simulink library "carnotUIBK"  (R2018b)
settings: Solver=VariableStepAuto  StartTime=0.0  StopTime=10.0  RelTol=1e-3  EnableMultiTasking=on
values from neighbouring files (symbols this model uses):
  A = 7*10*2    (= 140)    [theta_ground_v1.m]    (also in xlswrite1.m = num2cell(data))
  amb_factor = 1    [DOOR.m]    (also in WALL.m; WINDOW.m = 0)
  area = obj.width * obj.height    [DOOR.m]    (also in RES.m = []; ROOM.m = 0; THERMALZONE.m = area + room(kk).area; WALL.m = area - obj.doors(jj).calc_area())
  B = A/(0.5 * P)    (= 8.23529411765)    [theta_ground_v1.m]
  boundary = BOUNDARY()    [BUILDING.m]    (also in WALL.m = '')
  building = obj    [BUILDING.m]    (also in create_building_automatic.m = building.save(); ini_building_automatic.m = building.add_variant_hvac(building.variant_hvac, hvac); load_building_automatic.m = building.save())
  C = zeros(1,length(d)+1)    [CONSTRUCTION.m]    (also in DOOR.m = [0 0 0]; WALL.m = [0 0 0]; WINDOW.m = [0 0 0])
  control = 2    [GAIN.m]    (also in GAINS.m)
  cp = str2num(value)    [CONSTRUCTION.m]
  height = 0    [DOOR.m]    (also in ROOM.m; THERMALZONE.m; WALL.m; WINDOW.m)
  p = [timevec_weather weather(:,12)]    [BOUNDARY.m]    (also in WEATHER.m = 0; init_carnotUIBK.m = cell2mat(carnotUIBKpaths(i,2)))
  rho = str2num(value)    [CONSTRUCTION.m]    (also in theta_ground_v1.m = 2000)
  type = 1    [CONSTRUCTION.m]    (also in GAINS.m = raw_moisture{ii,3}; STRUCTURE.m = 0)
  view_factor = 1    [DOOR.m]    (also in WINDOW.m = 0)
  wall = []    [ROOM.m]
  z = obj.Z    [WALL.m]    (also in theta_ground_v1.m = 0)
  zone = obj.zone(ind)    [THERMALZONE.m]
undefined symbols (not defined in the file or in its folder): const, Dd, get_building, pos, Qdot_C, Qdot_H, Qdot_I_electricity, Qdot_I_light, Qdot_I_person, Qdot_S, Qdot_T_ground, Qdot_T_neighbour, Qdot_T_opaque, Qdot_T_window, Qdot_V_infiltration, Qdot_V_mech, Qdot_V_window, r_frame, solar_ratio, solar_ratio1, solar_ratio2, Tc, Tr, Ts, Uvalue, wallsurface, window, window_height, window_heigth, window_width, windowsurface, x_CO2, x_H2O, x_VOC
libraries: carnot x104, simulink x16, $bdroot x16, simulink_extras x14
(part 10 of 12)

== system carnotUIBK/wall_intersection/hygrothermal model/alpha_i2/alpha_i_horizontal ==
  note: (W/m^2)
  note: Convective and radiative heat transfer at the INDOOR SURFACE of a VERTICAL OUTER WALL
  note: CONVENTION:
      | Qdot > 0 and qdots < 0, if Ts > T (heat flows from wall surface to room node),
      | Qdot < 0 and qdots > 0, if Ts < T (heat flows from room node to wall surface).
  note: s: surface
      | c: convective
      | r: radiative
  note: dynamic, convective heat transfer coefficients according to: Glück B.: Wärmeübergangskoeffizienten an thermisch aktiven Bauteiloberflächen
      | und der Übergang zu Basiskennlinien für die Wärmestromdichte; gi Gesundheits-Ingenieur; 128. Jahrgang 2007, Heft 1, Seiten 1-10
  Ts : Inport
  AIB : Inport  Port=2
  Qdot sol : Inport  Port=3
  phis : Inport  Port=4
  1/wallsurface : Gain  Gain=1/wallsurface  SaturateOnIntegerOverflow=on  OutDataTypeStr=Inherit: Same as input  ParamDataTypeStr=Inherit: Same as input
  Add : Sum  Inputs=+-
  Bus Selector : BusSelector  OutputSignals=Tc,Tr,p,x_H2O
  Constant3 : Constant  Value=zeros(1,2)
  Constant4 : Constant  Value=zeros(1,4)
  Constant5 : Constant  Value=zeros(1,9)
  Fcn : Fcn  Expr=1.6*(abs(u(1)-u(2)))^0.3
  Fcn1 : Fcn  Expr=(273.15+u(1))^4-(273.15+u(2))^4
  Gain2 : Gain  Gain=0.01
  Mux : Mux  Inputs=2
  Mux2 : Mux  Inputs=2
  Mux3 : Mux  Inputs=2
  Mux4 : Mux  Inputs=[2 2 1 4 1 9]
  Product : Product  SaturateOnIntegerOverflow=on  RndMeth=Zero  InputSameDT=on  OutDataTypeStr=Inherit: Same as first input
  Product1 : Product  SaturateOnIntegerOverflow=on  RndMeth=Zero  InputSameDT=on  OutDataTypeStr=Inherit: Same as first input
  Product2 : Product  RndMeth=Zero
  Product3 : Product  RndMeth=Zero
  Product4 : Product  SaturateOnIntegerOverflow=on  RndMeth=Zero  InputSameDT=on  OutDataTypeStr=Inherit: Same as first input
  Sum : Sum  Inputs=+-  SaturateOnIntegerOverflow=on  InputSameDT=on  OutDataTypeStr=Inherit: Same as first input
  Sum of Elements : Sum  Inputs=+
  Sum2 : Sum  Inputs=+--  SaturateOnIntegerOverflow=on  InputSameDT=on  OutDataTypeStr=Inherit: Same as first input
  Switch : Switch  Criteria=u2 > Threshold
  emission_in : Gain  Gain=emission_in  SaturateOnIntegerOverflow=on  OutDataTypeStr=Inherit: Same as input  ParamDataTypeStr=Inherit: Same as input
  lewis : Gain  Gain=0.000000007  SaturateOnIntegerOverflow=on  OutDataTypeStr=Inherit: Same as input  ParamDataTypeStr=Inherit: Same as input
  nomassflow : Constant  Value=0
  ps_l : Fcn  Expr=610.0*exp(17.08*(u)/(234.2+(u)))
  ps_s_l : Fcn  Expr=610.0*exp(17.08*(u)/(234.2+(u)))
  sigma : Constant  Value=5.67e-8
  view_factor : Gain  Gain=view_factor  SaturateOnIntegerOverflow=on  OutDataTypeStr=Inherit: Same as input  ParamDataTypeStr=Inherit: Same as input
  wallsurface : Gain  Gain=wallsurface  SaturateOnIntegerOverflow=on  OutDataTypeStr=Inherit: Same as input  ParamDataTypeStr=Inherit: Same as input
  wallsurface1 : Gain  Gain=wallsurface  SaturateOnIntegerOverflow=on  OutDataTypeStr=Inherit: Same as input  ParamDataTypeStr=Inherit: Same as input
  x2RelHum_UIBK : carnot/Basic/Material_Properties/x2RelHum
  qdots : Outport  InitialOutput=0
  "[S]" : Outport  Port=2  InitialOutput=0
  alpha_c : Outport  Port=3  InitialOutput=0
  phi_i_1/100 : Outport  Port=4  InitialOutput=0
  wires:
  nomassflow/1 -> Switch/3
  Switch/1 -> Mux4/3
  wallsurface1/1 -> Switch/1
  view_factor/1 -> Product/1
  phis/1 -> Product3/1, Switch/2
  Product2/1 -> Add/2
  Product3/1 -> Add/1
  ps_s_l/1 -> Product3/2
  ps_l/1 -> Product2/2
  lewis/1 -> wallsurface1/1
  Gain2/1 -> Product2/1, phi_i_1/100/1
  Bus Selector/4 -> x2RelHum_UIBK/3  "<x_H2O>"
  Bus Selector/3 -> x2RelHum_UIBK/2  "<p>"
  x2RelHum_UIBK/1 -> Gain2/1
  Fcn1/1 -> Product/2
  Mux3/1 -> Fcn1/1
  sigma/1 -> emission_in/1
  Mux4/1 -> "[S]"/1
  Sum2/1 -> qdots/1
  AIB/1 -> Bus Selector/1
  Bus Selector/1 -> Sum/2, Mux2/2, x2RelHum_UIBK/1, ps_l/1  "<Tc>"
  emission_in/1 -> view_factor/1
  Product/1 -> Sum2/3, Mux/2  "qdotr"
  Mux/1 -> wallsurface/1
  Ts/1 -> Sum/1, ps_s_l/1, Mux3/1, Mux2/1  "Ts"
  Sum/1 -> Product1/1  "dTc"
  Bus Selector/2 -> Mux3/2  "<Tr>"
  Mux2/1 -> Fcn/1
  Product1/1 -> Mux/1, Sum2/2  "qdotc"
  Fcn/1 -> Product4/1, alpha_c/1, Product1/2  "hc"
  wallsurface/1 -> Sum of Elements/1, Mux4/1  "[Qdotc, Qdotr]"
  Qdot sol/1 -> 1/wallsurface/1
  1/wallsurface/1 -> Sum2/1
  Constant5/1 -> Mux4/6
  Constant4/1 -> Mux4/4
  Constant3/1 -> Mux4/2
  Sum of Elements/1 -> Mux4/5
  Add/1 -> Product4/2
  Product4/1 -> lewis/1

== system carnotUIBK/wall_intersection/hygrothermal model/alpha_i2/alpha_i_up ==
  note: (W/m^2)
  note: Convective and radiative heat transfer at the INDOOR SURFACE of a ceiling
  note: CONVENTION:
      | Qdot > 0 and qdots < 0, if Ts > T (heat flows from wall surface to room node),
      | Qdot < 0 and qdots > 0, if Ts < T (heat flows from room node to wall surface).
  note: s: surface
      | c: convective
      | r: radiative
  note: dynamic, convective heat transfer coefficients according to: Glück B.: Wärmeübergangskoeffizienten an thermisch aktiven Bauteiloberflächen
      | und der Übergang zu Basiskennlinien für die Wärmestromdichte; gi Gesundheits-Ingenieur; 128. Jahrgang 2007, Heft 1, Seiten 1-10
  Ts : Inport
  AIB : Inport  Port=2
  Qdot sol : Inport  Port=3
  phis : Inport  Port=4
  1/wallsurface : Gain  Gain=1/wallsurface  SaturateOnIntegerOverflow=on  OutDataTypeStr=Inherit: Same as input  ParamDataTypeStr=Inherit: Same as input
  Add : Sum  Inputs=+-
  Bus Selector : BusSelector  OutputSignals=Tc,Tr,p,x_H2O
  Constant3 : Constant  Value=zeros(1,2)
  Constant4 : Constant  Value=zeros(1,4)
  Constant5 : Constant  Value=zeros(1,9)
  Fcn1 : Fcn  Expr=(273.15+u(1))^4-(273.15+u(2))^4
  Gain2 : Gain  Gain=0.01
  Mux : Mux  Inputs=2
  Mux2 : Mux  Inputs=2
  Mux3 : Mux  Inputs=2
  Mux4 : Mux  Inputs=[2 2 1 4 1 9]
  Product : Product  SaturateOnIntegerOverflow=on  RndMeth=Zero  InputSameDT=on  OutDataTypeStr=Inherit: Same as first input
  Product1 : Product  SaturateOnIntegerOverflow=on  RndMeth=Zero  InputSameDT=on  OutDataTypeStr=Inherit: Same as first input
  Product2 : Product  RndMeth=Zero
  Product3 : Product  RndMeth=Zero
  Product4 : Product  SaturateOnIntegerOverflow=on  RndMeth=Zero  InputSameDT=on  OutDataTypeStr=Inherit: Same as first input
  Sum : Sum  Inputs=+-  SaturateOnIntegerOverflow=on  InputSameDT=on  OutDataTypeStr=Inherit: Same as first input
  Sum of Elements : Sum  Inputs=+
  Sum2 : Sum  Inputs=+--  SaturateOnIntegerOverflow=on  InputSameDT=on  OutDataTypeStr=Inherit: Same as first input
  Switch : Switch  Criteria=u2 > Threshold
  Switch1 : Switch
  emission_in : Gain  Gain=emission_in  SaturateOnIntegerOverflow=on  OutDataTypeStr=Inherit: Same as input  ParamDataTypeStr=Inherit: Same as input
  heat flux downwards : Fcn  Expr=0.54*(abs(u(1)-u(2))^0.31)
  heat flux upwards : Fcn  Expr=2*(abs(u(1)-u(2))^0.31)
  lewis : Gain  Gain=0.000000007  SaturateOnIntegerOverflow=on  OutDataTypeStr=Inherit: Same as input  ParamDataTypeStr=Inherit: Same as input
  nomassflow : Constant  Value=0
  ps_l : Fcn  Expr=610.0*exp(17.08*(u)/(234.2+(u)))
  ps_s_l : Fcn  Expr=610.0*exp(17.08*(u)/(234.2+(u)))
  sigma : Constant  Value=5.67e-8
  view_factor : Gain  Gain=view_factor  SaturateOnIntegerOverflow=on  OutDataTypeStr=Inherit: Same as input  ParamDataTypeStr=Inherit: Same as input
  wallsurface : Gain  Gain=wallsurface  SaturateOnIntegerOverflow=on  OutDataTypeStr=Inherit: Same as input  ParamDataTypeStr=Inherit: Same as input
  wallsurface1 : Gain  Gain=wallsurface  SaturateOnIntegerOverflow=on  OutDataTypeStr=Inherit: Same as input  ParamDataTypeStr=Inherit: Same as input
  x2RelHum_UIBK : carnot/Basic/Material_Properties/x2RelHum
  qdots : Outport  InitialOutput=0
  "[S]" : Outport  Port=2  InitialOutput=0
  alpha_c : Outport  Port=3  InitialOutput=0
  phi_i_1/100 : Outport  Port=4  InitialOutput=0
  wires:
  nomassflow/1 -> Switch/3
  Switch/1 -> Mux4/3
  wallsurface1/1 -> Switch/1
  view_factor/1 -> Product/1
  phis/1 -> Product3/1, Switch/2
  Product2/1 -> Add/2
  Product3/1 -> Add/1
  ps_s_l/1 -> Product3/2
  ps_l/1 -> Product2/2
  lewis/1 -> wallsurface1/1
  Gain2/1 -> Product2/1, phi_i_1/100/1
  Bus Selector/4 -> x2RelHum_UIBK/3  "<x_H2O>"
  Bus Selector/3 -> x2RelHum_UIBK/2  "<p>"
  x2RelHum_UIBK/1 -> Gain2/1
  Fcn1/1 -> Product/2
  Mux3/1 -> Fcn1/1
  sigma/1 -> emission_in/1
  Mux4/1 -> "[S]"/1
  Sum2/1 -> qdots/1
  AIB/1 -> Bus Selector/1
  Bus Selector/1 -> Sum/2, Mux2/2, x2RelHum_UIBK/1, ps_l/1  "<Tc>"
  emission_in/1 -> view_factor/1
  Product/1 -> Sum2/3, Mux/2  "qdotr"
  Mux/1 -> wallsurface/1
  Ts/1 -> Sum/1, ps_s_l/1, Mux3/1, Mux2/1  "Ts"
  Bus Selector/2 -> Mux3/2  "<Tr>"
  Mux2/1 -> heat flux downwards/1, heat flux upwards/1
  Product1/1 -> Mux/1, Sum2/2  "qdotc"
  Switch1/1 -> Product1/2, Product4/1, alpha_c/1  "hc"
  wallsurface/1 -> Sum of Elements/1, Mux4/1  "[Qdotc, Qdotr]"
  Qdot sol/1 -> 1/wallsurface/1
  1/wallsurface/1 -> Sum2/1
  Sum/1 -> Switch1/2, Product1/1  "dTc"
  heat flux upwards/1 -> Switch1/3
  heat flux downwards/1 -> Switch1/1
  Constant5/1 -> Mux4/6
  Constant4/1 -> Mux4/4
  Constant3/1 -> Mux4/2
  Sum of Elements/1 -> Mux4/5
  Product4/1 -> lewis/1
  Add/1 -> Product4/2

== system carnotUIBK/wall_zone/R-C model/alpha_e/alpha_e_AMBIENT ==
  note: dynamic, convective heat transfer coefficients according to: Glück B.: Wärmeübergangskoeffizienten an thermisch aktiven Bauteiloberflächen
      | und der Übergang zu Basiskennlinien für die Wärmestromdichte; gi Gesundheits-Ingenieur; 128. Jahrgang 2007, Heft 1, Seiten 1-10
  note: Convective heat transfer outer surface according to EN 6946
      | Radiative heat transfer to the ground is limited by a view of 0.25, i.e. view factor to the sky is 0.75 (Frohner, 2005)
  note: s: surface
      | c: convective
      | r: radiative
      | h: in height
      | t: tilted surface
  note: CONVENTION:
      | qdots < 0, if Ts > T, heat flows from window surface (resp. room node) to ambient,
      | qdots > 0, if Ts < T, heat flows from ambient to window surface (resp. room node).
  WDB : Inport
  GDB : Inport  Port=2
  NDB : Inport  Port=3
  AIB : Inport  Port=4
  Ts : Inport  Port=5
  Qdot_sol : Inport  Port=6
  phis : Inport  Port=7
  1/100 : Gain  Gain=1/100
  Bus Selector : BusSelector  OutputSignals=Temperature_Ambient,Temperature_Sky_Radiation,Wind_Speed,Relative_Humidity
  Constant : Constant  Value=zeros(1,5)
  Constant1 : Constant  Value=zeros(1,2)
  Constant2 : Constant  Value=zeros(1,9)
  Mux1 : Mux  Inputs=[1 1 5 1 2 9]
  Product2 : Product  SaturateOnIntegerOverflow=on  RndMeth=Zero  InputSameDT=on  OutDataTypeStr=Inherit: Same as first input
  Qdotc : Constant  Value=0
  Qdotr : Constant  Value=0
  Sum : Sum  Inputs=+-  SaturateOnIntegerOverflow=on  InputSameDT=on  OutDataTypeStr=Inherit: Same as first input
  Sum2 : Sum  Inputs=+++  SaturateOnIntegerOverflow=on  InputSameDT=on  OutDataTypeStr=Inherit: Same as first input
  Terminator{,1..4} (5 alike) : Terminator
  absorption_out : Gain  Gain=absorption_out  SaturateOnIntegerOverflow=on  OutDataTypeStr=Inherit: Same as input  ParamDataTypeStr=Inherit: Same as input
  qp rad : Subsystem
  wall_surfrad : Subsystem  mask{pos=pos}
      mask prompts: pos "Position"
  wallsurface : Gain  Gain=wallsurface  SaturateOnIntegerOverflow=on  OutDataTypeStr=Inherit: Same as input  ParamDataTypeStr=Inherit: Same as input
  wind dependent heat transfer EN 6946 : Fcn  Expr=4*u(1)+4
  qdots : Outport  InitialOutput=0
  "[S]" : Outport  Port=2  InitialOutput=0
  alpha_c : Outport  Port=3  InitialOutput=0
  phi_e_1/100 : Outport  Port=4  InitialOutput=0
  theta_e : Outport  Port=5  InitialOutput=0
  wires:
  wallsurface/1 -> Mux1/4
  Sum2/1 -> qdots/1, wallsurface/1
  Qdotr/1 -> Mux1/2
  Qdotc/1 -> Mux1/1
  Constant/1 -> Mux1/3
  Constant1/1 -> Mux1/5
  Constant2/1 -> Mux1/6
  Mux1/1 -> "[S]"/1
  NDB/1 -> Terminator1/1
  GDB/1 -> Terminator/1
  Bus Selector/3 -> wind dependent heat transfer EN 6946/1  "<Wind_Speed>"
  Bus Selector/2 -> qp rad/3(Tsky)  "<Temperature_Sky_Radiation>"
  Bus Selector/1 -> theta_e/1, qp rad/1(Ta), Sum/1  "<Temperature_Ambient>"
  Sum/1 -> Product2/1  "dTc"
  WDB/1 -> wall_surfrad/1(WDB), Bus Selector/1
  Ts/1 -> Sum/2, qp rad/2(Tw)  "Ts (outer wall surface)"
  wall_surfrad/1(Idir,t+Idfu,t) -> absorption_out/1
  wind dependent heat transfer EN 6946/1 -> Product2/2, alpha_c/1  "alfa"
  absorption_out/1 -> Sum2/3  "qdot,sun"
  Product2/1 -> Sum2/1  "qdotc"
  qp rad/1(qprad) -> Sum2/2  "qdotr"
  AIB/1 -> Terminator2/1
  Qdot_sol/1 -> Terminator3/1
  phis/1 -> Terminator4/1
  Bus Selector/4 -> 1/100/1  "<Relative_Humidity>"
  1/100/1 -> phi_e_1/100/1

== system carnotUIBK/wall_zone/R-C model/alpha_e/alpha_e_GROUND ==
  note: dynamic, convective heat transfer coefficients according to: Glück B.: Wärmeübergangskoeffizienten an thermisch aktiven Bauteiloberflächen
      | und der Übergang zu Basiskennlinien für die Wärmestromdichte; gi Gesundheits-Ingenieur; 128. Jahrgang 2007, Heft 1, Seiten 1-10
  note: Convective heat transfer outer surface according to EN 6946
      | Radiative heat transfer to the ground is limited by a view of 0.25, i.e. view factor to the sky is 0.75 (Frohner, 2005)
  note: s: surface
      | c: convective
      | r: radiative
      | h: in height
      | t: tilted surface
  note: CONVENTION:
      | qdots < 0, if Ts > T, heat flows from window surface (resp. room node) to ambient,
      | qdots > 0, if Ts < T, heat flows from ambient to window surface (resp. room node).
  WDB : Inport
  GDB : Inport  Port=2
  NDB : Inport  Port=3
  AIB : Inport  Port=4
  Ts : Inport  Port=5
  Qdot_sol : Inport  Port=6
  phis : Inport  Port=7
  Constant : Constant  Value=zeros(1,5)
  Constant1 : Constant  Value=0
  Constant2 : Constant  Value=zeros(1,10)
  Mux1 : Mux  Inputs=[1 1 5 1 1 10]
  Qdotc : Constant  Value=0
  Qdotr : Constant  Value=0
  Sum : Sum  Inputs=+-  SaturateOnIntegerOverflow=on  InputSameDT=on  OutDataTypeStr=Inherit: Same as first input
  Terminator{,1..4} (5 alike) : Terminator
  alpha1000 : Constant  Value=1000
  alpha_ground : Gain  Gain=1000
  phi100 : Constant
  wallsurface : Gain  Gain=wallsurface  SaturateOnIntegerOverflow=on  OutDataTypeStr=Inherit: Same as input  ParamDataTypeStr=Inherit: Same as input
  qdots : Outport  InitialOutput=0
  "[S]" : Outport  Port=2  InitialOutput=0
  alpha_c : Outport  Port=3  InitialOutput=0
  phi_e_1/100 : Outport  Port=4  InitialOutput=0
  theta_e : Outport  Port=5  InitialOutput=0
  wires:
  alpha_ground/1 -> qdots/1, wallsurface/1
  Qdotr/1 -> Mux1/2
  Qdotc/1 -> Mux1/1
  Constant/1 -> Mux1/3
  Constant2/1 -> Mux1/6
  Mux1/1 -> "[S]"/1
  NDB/1 -> Terminator1/1
  GDB/1 -> theta_e/1, Sum/1
  Sum/1 -> alpha_ground/1  "dT"
  Ts/1 -> Sum/2  "Ts (outer wall surface)"
  AIB/1 -> Terminator2/1
  WDB/1 -> Terminator/1
  Qdot_sol/1 -> Terminator3/1
  phis/1 -> Terminator4/1
  phi100/1 -> phi_e_1/100/1
  alpha1000/1 -> alpha_c/1
  Constant1/1 -> Mux1/4
  wallsurface/1 -> Mux1/5

== system carnotUIBK/wall_zone/R-C model/alpha_e/alpha_e_INTERNAL ==
  note: dynamic, convective heat transfer coefficients according to: Glück B.: Wärmeübergangskoeffizienten an thermisch aktiven Bauteiloberflächen
      | und der Übergang zu Basiskennlinien für die Wärmestromdichte; gi Gesundheits-Ingenieur; 128. Jahrgang 2007, Heft 1, Seiten 1-10
  note: Convective heat transfer outer surface according to EN 6946
      | Radiative heat transfer to the ground is limited by a view of 0.25, i.e. view factor to the sky is 0.75 (Frohner, 2005)
  note: s: surface
      | c: convective
      | r: radiative
      | h: in height
      | t: tilted surface
  note: CONVENTION:
      | qdots < 0, if Ts > T, heat flows from window surface (resp. room node) to ambient,
      | qdots > 0, if Ts < T, heat flows from ambient to window surface (resp. room node).
  WDB : Inport
  GDB : Inport  Port=2
  NDB : Inport  Port=3
  AIB : Inport  Port=4
  Ts : Inport  Port=5
  Qdot_sol : Inport  Port=6
  phis : Inport  Port=7
  Bus Selector : BusSelector  OutputSignals=Tc
  Terminator : Terminator
  Terminator1 : Terminator
  Terminator2 : Terminator
  alpha_i : Subsystem  Variant=on  mask{view_factor=amb_factor}
  qdots : Outport  InitialOutput=0
  "[S]" : Outport  Port=2  InitialOutput=0
  alpha_c : Outport  Port=3  InitialOutput=0
  phi_e_1/100 : Outport  Port=4  InitialOutput=0
  theta_e : Outport  Port=5  InitialOutput=0
  wires:
  NDB/1 -> Terminator1/1
  GDB/1 -> Terminator/1
  WDB/1 -> Terminator2/1
  Ts/1 -> alpha_i/1(Ts)  "Ts (outer wall surface)"
  Qdot_sol/1 -> alpha_i/3(Qdot sol)
  alpha_i/1(qdots) -> qdots/1
  alpha_i/3(alpha_c) -> alpha_c/1
  alpha_i/2("[S]") -> "[S]"/1
  AIB/1 -> alpha_i/2(AIB), Bus Selector/1
  phis/1 -> alpha_i/4(phis)
  alpha_i/4(phi_i_1/100) -> phi_e_1/100/1
  Bus Selector/1 -> theta_e/1  "<Tc>"

== system carnotUIBK/wall_zone/R-C model/alpha_e/alpha_e_NEIGHBOUR ==
  note: dynamic, convective heat transfer coefficients according to: Glück B.: Wärmeübergangskoeffizienten an thermisch aktiven Bauteiloberflächen
      | und der Übergang zu Basiskennlinien für die Wärmestromdichte; gi Gesundheits-Ingenieur; 128. Jahrgang 2007, Heft 1, Seiten 1-10
  note: Convective heat transfer outer surface according to EN 6946
      | Radiative heat transfer to the ground is limited by a view of 0.25, i.e. view factor to the sky is 0.75 (Frohner, 2005)
  note: s: surface
      | c: convective
      | r: radiative
      | h: in height
      | t: tilted surface
  note: CONVENTION:
      | qdots < 0, if Ts > T, heat flows from window surface (resp. room node) to ambient,
      | qdots > 0, if Ts < T, heat flows from ambient to window surface (resp. room node).
  WDB : Inport
  GDB : Inport  Port=2
  NDB : Inport  Port=3
  AIB : Inport  Port=4
  Ts : Inport  Port=5
  Qdot_sol : Inport  Port=6
  phis : Inport  Port=7
  Demux : Demux  Outputs=[2 5 1 1 10]
  Mux1 : Mux  Inputs=[1 1 5 1 1 10]
  Qdot sol neighbour : Constant  Value=0
  Qdot_T_opaque : Constant  Value=0
  Qdot_c : Constant  Value=0
  Qdot_r : Constant  Value=0
  Terminator{,1..4} (5 alike) : Terminator
  alpha_i : Subsystem  Variant=on  mask{view_factor=1}
  set temperature : BusAssignment  AssignedSignals=Ts,Tc,Tr
  qdots : Outport  InitialOutput=0
  "[S]" : Outport  Port=2  InitialOutput=0
  alpha_c : Outport  Port=3  InitialOutput=0
  phi_e_1/100 : Outport  Port=4  InitialOutput=0
  theta_e : Outport  Port=5  InitialOutput=0
  wires:
  GDB/1 -> Terminator/1
  WDB/1 -> Terminator2/1
  Ts/1 -> alpha_i/1(Ts)  "Ts (outer wall surface)"
  alpha_i/1(qdots) -> qdots/1
  alpha_i/3(alpha_c) -> alpha_c/1
  phis/1 -> alpha_i/4(phis)
  alpha_i/4(phi_i_1/100) -> phi_e_1/100/1
  Qdot_sol/1 -> Terminator3/1
  Qdot sol neighbour/1 -> alpha_i/3(Qdot sol)
  AIB/1 -> set temperature/1
  NDB/1 -> theta_e/1, set temperature/4, set temperature/3, set temperature/2
  set temperature/1 -> alpha_i/2(AIB)
  alpha_i/2("[S]") -> Demux/1
  Demux/2 -> Mux1/3
  Demux/5 -> Mux1/6
  Mux1/1 -> "[S]"/1
  Qdot_T_opaque/1 -> Mux1/4
  Demux/3 -> Terminator4/1
  Demux/4 -> Mux1/5
  Demux/1 -> Terminator1/1
  Qdot_c/1 -> Mux1/1
  Qdot_r/1 -> Mux1/2

== system carnotUIBK/wall_zone/R-C model/alpha_i/alpha_i_down ==
  note: (W/m^2)
  note: Convective and radiative heat transfer at the INDOOR SURFACE of a floor
  note: CONVENTION:
      | Qdot > 0 and qdots < 0, if Ts > T (heat flows from wall surface to room node),
      | Qdot < 0 and qdots > 0, if Ts < T (heat flows from room node to wall surface).
  note: s: surface
      | c: convective
      | r: radiative
  note: dynamic, convective heat transfer coefficients according to: Glück B.: Wärmeübergangskoeffizienten an thermisch aktiven Bauteiloberflächen
      | und der Übergang zu Basiskennlinien für die Wärmestromdichte; gi Gesundheits-Ingenieur; 128. Jahrgang 2007, Heft 1, Seiten 1-10
  Ts : Inport
  AIB : Inport  Port=2
  Qdot sol : Inport  Port=3
  phis : Inport  Port=4
  1/wallsurface : Gain  Gain=1/wallsurface  SaturateOnIntegerOverflow=on  OutDataTypeStr=Inherit: Same as input  ParamDataTypeStr=Inherit: Same as input
  Add : Sum  Commented=on  Inputs=+-
  Bus Selector : BusSelector  OutputSignals=Tc,Tr,p,x_H2O
  Constant : Constant  Value=zeros(1,2)
  Constant1 : Constant  Value=zeros(1,2)
  Constant2 : Constant  Value=zeros(1,12)
  Fcn1 : Fcn  Expr=(273.15+u(1))^4-(273.15+u(2))^4
  Gain2 : Gain  Commented=on  Gain=0.01
  Mux : Mux  Inputs=2
  Mux1 : Mux  Inputs=[2 2 1 2 12]
  Mux2 : Mux  Inputs=2
  Mux3 : Mux  Inputs=2
  Product : Product  SaturateOnIntegerOverflow=on  RndMeth=Zero  InputSameDT=on  OutDataTypeStr=Inherit: Same as first input
  Product1 : Product  SaturateOnIntegerOverflow=on  RndMeth=Zero  InputSameDT=on  OutDataTypeStr=Inherit: Same as first input
  Product2 : Product  Commented=on  RndMeth=Zero
  Product3 : Product  Commented=on  RndMeth=Zero
  Sum : Sum  Inputs=+-  SaturateOnIntegerOverflow=on  InputSameDT=on  OutDataTypeStr=Inherit: Same as first input
  Sum2 : Sum  Inputs=+--  SaturateOnIntegerOverflow=on  InputSameDT=on  OutDataTypeStr=Inherit: Same as first input
  Switch : Switch  Commented=on  Criteria=u2 > Threshold
  Switch1 : Switch
  emission_in : Gain  Gain=emission_in  SaturateOnIntegerOverflow=on  OutDataTypeStr=Inherit: Same as input  ParamDataTypeStr=Inherit: Same as input
  heat flux downwards : Fcn  Expr=0.54*(abs(u(1)-u(2))^0.31)
  heat flux upwards : Fcn  Expr=2*(abs(u(1)-u(2))^0.31)
  lewis : Gain  Commented=on  Gain=0.000000007  SaturateOnIntegerOverflow=on  OutDataTypeStr=Inherit: Same as input  ParamDataTypeStr=Inherit: Same as input
  nomassflow : Constant  Value=0
  ps_l : Fcn  Commented=on  Expr=610.0*exp(17.08*(u)/(234.2+(u)))
  ps_s_l : Fcn  Commented=on  Expr=610.0*exp(17.08*(u)/(234.2+(u)))
  sigma : Constant  Value=5.67e-8
  view_factor : Gain  Gain=view_factor  SaturateOnIntegerOverflow=on  OutDataTypeStr=Inherit: Same as input  ParamDataTypeStr=Inherit: Same as input
  wallsurface : Gain  Gain=wallsurface  SaturateOnIntegerOverflow=on  OutDataTypeStr=Inherit: Same as input  ParamDataTypeStr=Inherit: Same as input
  wallsurface1 : Gain  Commented=on  Gain=wallsurface  SaturateOnIntegerOverflow=on  OutDataTypeStr=Inherit: Same as input  ParamDataTypeStr=Inherit: Same as input
  x2RelHum_UIBK : carnot/Basic/Material_Properties/x2RelHum  Commented=on
  qdots : Outport  InitialOutput=0
  "[S]" : Outport  Port=2  InitialOutput=0
  alpha_c : Outport  Port=3  InitialOutput=0
  phi_i_1/100 : Outport  Port=4  InitialOutput=0
  wires:
  nomassflow/1 -> Mux1/3, Switch/3
  wallsurface1/1 -> Switch/1
  view_factor/1 -> Product/1
  phis/1 -> Product3/1, Switch/2
  Add/1 -> lewis/1
  Product2/1 -> Add/2
  Product3/1 -> Add/1
  ps_s_l/1 -> Product3/2
  ps_l/1 -> Product2/2
  Constant/1 -> Mux1/2
  Constant1/1 -> Mux1/4
  Constant2/1 -> Mux1/5
  lewis/1 -> wallsurface1/1
  Gain2/1 -> Product2/1, phi_i_1/100/1
  Bus Selector/4 -> x2RelHum_UIBK/3  "<x_H2O>"
  Bus Selector/3 -> x2RelHum_UIBK/2  "<p>"
  x2RelHum_UIBK/1 -> Gain2/1
  Fcn1/1 -> Product/2
  Mux3/1 -> Fcn1/1
  sigma/1 -> emission_in/1
  Mux1/1 -> "[S]"/1
  Sum2/1 -> qdots/1
  AIB/1 -> Bus Selector/1
  Bus Selector/1 -> Sum/2, Mux2/2, x2RelHum_UIBK/1, ps_l/1  "<Tc>"
  emission_in/1 -> view_factor/1
  Product/1 -> Sum2/3, Mux/2  "qdotr"
  Mux/1 -> wallsurface/1
  Ts/1 -> Sum/1, ps_s_l/1, Mux3/1, Mux2/1  "Ts"
  Bus Selector/2 -> Mux3/2  "<Tr>"
  Mux2/1 -> heat flux downwards/1, heat flux upwards/1
  Product1/1 -> Mux/1, Sum2/2  "qdotc"
  Switch1/1 -> Product1/2, alpha_c/1  "hc"
  wallsurface/1 -> Mux1/1  "[Qdotc, Qdotr]"
  Qdot sol/1 -> 1/wallsurface/1
  1/wallsurface/1 -> Sum2/1
  Sum/1 -> Switch1/2, Product1/1  "dTc"
  heat flux upwards/1 -> Switch1/1
  heat flux downwards/1 -> Switch1/3

== system carnotUIBK/wall_zone/R-C model/alpha_i/alpha_i_horizontal ==
  note: (W/m^2)
  note: Convective and radiative heat transfer at the INDOOR SURFACE of a VERTICAL OUTER WALL
  note: CONVENTION:
      | Qdot > 0 and qdots < 0, if Ts > T (heat flows from wall surface to room node),
      | Qdot < 0 and qdots > 0, if Ts < T (heat flows from room node to wall surface).
  note: s: surface
      | c: convective
      | r: radiative
  note: dynamic, convective heat transfer coefficients according to: Glück B.: Wärmeübergangskoeffizienten an thermisch aktiven Bauteiloberflächen
      | und der Übergang zu Basiskennlinien für die Wärmestromdichte; gi Gesundheits-Ingenieur; 128. Jahrgang 2007, Heft 1, Seiten 1-10
  Ts : Inport
  AIB : Inport  Port=2
  Qdot sol : Inport  Port=3
  phis : Inport  Port=4
  1/wallsurface : Gain  Gain=1/wallsurface  SaturateOnIntegerOverflow=on  OutDataTypeStr=Inherit: Same as input  ParamDataTypeStr=Inherit: Same as input
  Add : Sum  Commented=on  Inputs=+-
  Bus Selector : BusSelector  OutputSignals=Tc,Tr,p,x_H2O
  Constant : Constant  Value=zeros(1,2)
  Constant1 : Constant  Value=zeros(1,2)
  Constant2 : Constant  Value=zeros(1,12)
  Fcn : Fcn  Expr=1.6*(abs(u(1)-u(2)))^0.3
  Fcn1 : Fcn  Expr=(273.15+u(1))^4-(273.15+u(2))^4
  Gain2 : Gain  Commented=on  Gain=0.01
  Mux : Mux  Inputs=2
  Mux1 : Mux  Inputs=[2 2 1 2 12]
  Mux2 : Mux  Inputs=2
  Mux3 : Mux  Inputs=2
  Product : Product  SaturateOnIntegerOverflow=on  RndMeth=Zero  InputSameDT=on  OutDataTypeStr=Inherit: Same as first input
  Product1 : Product  SaturateOnIntegerOverflow=on  RndMeth=Zero  InputSameDT=on  OutDataTypeStr=Inherit: Same as first input
  Product2 : Product  Commented=on  RndMeth=Zero
  Product3 : Product  Commented=on  RndMeth=Zero
  Sum : Sum  Inputs=+-  SaturateOnIntegerOverflow=on  InputSameDT=on  OutDataTypeStr=Inherit: Same as first input
  Sum2 : Sum  Inputs=+--  SaturateOnIntegerOverflow=on  InputSameDT=on  OutDataTypeStr=Inherit: Same as first input
  Switch : Switch  Commented=on  Criteria=u2 > Threshold
  emission_in : Gain  Gain=emission_in  SaturateOnIntegerOverflow=on  OutDataTypeStr=Inherit: Same as input  ParamDataTypeStr=Inherit: Same as input
  lewis : Gain  Commented=on  Gain=0.000000007  SaturateOnIntegerOverflow=on  OutDataTypeStr=Inherit: Same as input  ParamDataTypeStr=Inherit: Same as input
  nomassflow : Constant  Value=0
  ps_l : Fcn  Commented=on  Expr=610.0*exp(17.08*(u)/(234.2+(u)))
  ps_s_l : Fcn  Commented=on  Expr=610.0*exp(17.08*(u)/(234.2+(u)))
  sigma : Constant  Value=5.67e-8
  view_factor : Gain  Gain=view_factor  SaturateOnIntegerOverflow=on  OutDataTypeStr=Inherit: Same as input  ParamDataTypeStr=Inherit: Same as input
  wallsurface : Gain  Gain=wallsurface  SaturateOnIntegerOverflow=on  OutDataTypeStr=Inherit: Same as input  ParamDataTypeStr=Inherit: Same as input
  wallsurface1 : Gain  Commented=on  Gain=wallsurface  SaturateOnIntegerOverflow=on  OutDataTypeStr=Inherit: Same as input  ParamDataTypeStr=Inherit: Same as input
  x2RelHum_UIBK : carnot/Basic/Material_Properties/x2RelHum  Commented=on
  qdots : Outport  InitialOutput=0
  "[S]" : Outport  Port=2  InitialOutput=0
  alpha_c : Outport  Port=3  InitialOutput=0
  phi_i_1/100 : Outport  Port=4  InitialOutput=0
  wires:
  nomassflow/1 -> Mux1/3, Switch/3
  wallsurface1/1 -> Switch/1
  view_factor/1 -> Product/1
  phis/1 -> Product3/1, Switch/2
  Add/1 -> lewis/1
  Product2/1 -> Add/2
  Product3/1 -> Add/1
  ps_s_l/1 -> Product3/2
  ps_l/1 -> Product2/2
  Constant/1 -> Mux1/2
  Constant1/1 -> Mux1/4
  Constant2/1 -> Mux1/5
  lewis/1 -> wallsurface1/1
  Gain2/1 -> Product2/1, phi_i_1/100/1
  Bus Selector/4 -> x2RelHum_UIBK/3  "<x_H2O>"
  Bus Selector/3 -> x2RelHum_UIBK/2  "<p>"
  x2RelHum_UIBK/1 -> Gain2/1
  Fcn1/1 -> Product/2
  Mux3/1 -> Fcn1/1
  sigma/1 -> emission_in/1
  Mux1/1 -> "[S]"/1
  Sum2/1 -> qdots/1
  AIB/1 -> Bus Selector/1
  Bus Selector/1 -> Sum/2, Mux2/2, x2RelHum_UIBK/1, ps_l/1  "<Tc>"
  emission_in/1 -> view_factor/1
  Product/1 -> Sum2/3, Mux/2  "qdotr"
  Mux/1 -> wallsurface/1
  Ts/1 -> Sum/1, ps_s_l/1, Mux3/1, Mux2/1  "Ts"
  Sum/1 -> Product1/1  "dTc"
  Bus Selector/2 -> Mux3/2  "<Tr>"
  Mux2/1 -> Fcn/1
  Product1/1 -> Mux/1, Sum2/2  "qdotc"
  Fcn/1 -> alpha_c/1, Product1/2  "hc"
  wallsurface/1 -> Mux1/1  "[Qdotc, Qdotr]"
  Qdot sol/1 -> 1/wallsurface/1
  1/wallsurface/1 -> Sum2/1

== system carnotUIBK/wall_zone/R-C model/alpha_i/alpha_i_up ==
  note: (W/m^2)
  note: Convective and radiative heat transfer at the INDOOR SURFACE of a ceiling
  note: CONVENTION:
      | Qdot > 0 and qdots < 0, if Ts > T (heat flows from wall surface to room node),
      | Qdot < 0 and qdots > 0, if Ts < T (heat flows from room node to wall surface).
  note: s: surface
      | c: convective
      | r: radiative
  note: dynamic, convective heat transfer coefficients according to: Glück B.: Wärmeübergangskoeffizienten an thermisch aktiven Bauteiloberflächen
      | und der Übergang zu Basiskennlinien für die Wärmestromdichte; gi Gesundheits-Ingenieur; 128. Jahrgang 2007, Heft 1, Seiten 1-10
  Ts : Inport
  AIB : Inport  Port=2
  Qdot sol : Inport  Port=3
  phis : Inport  Port=4
  1/wallsurface : Gain  Gain=1/wallsurface  SaturateOnIntegerOverflow=on  OutDataTypeStr=Inherit: Same as input  ParamDataTypeStr=Inherit: Same as input
  Add : Sum  Commented=on  Inputs=+-
  Bus Selector : BusSelector  OutputSignals=Tc,Tr,p,x_H2O
  Constant : Constant  Value=zeros(1,2)
  Constant1 : Constant  Value=zeros(1,2)
  Constant2 : Constant  Value=zeros(1,12)
  Fcn1 : Fcn  Expr=(273.15+u(1))^4-(273.15+u(2))^4
  Gain2 : Gain  Commented=on  Gain=0.01
  Mux : Mux  Inputs=2
  Mux1 : Mux  Inputs=[2 2 1 2 12]
  Mux2 : Mux  Inputs=2
  Mux3 : Mux  Inputs=2
  Product : Product  SaturateOnIntegerOverflow=on  RndMeth=Zero  InputSameDT=on  OutDataTypeStr=Inherit: Same as first input
  Product1 : Product  SaturateOnIntegerOverflow=on  RndMeth=Zero  InputSameDT=on  OutDataTypeStr=Inherit: Same as first input
  Product2 : Product  Commented=on  RndMeth=Zero
  Product3 : Product  Commented=on  RndMeth=Zero
  Sum : Sum  Inputs=+-  SaturateOnIntegerOverflow=on  InputSameDT=on  OutDataTypeStr=Inherit: Same as first input
  Sum2 : Sum  Inputs=+--  SaturateOnIntegerOverflow=on  InputSameDT=on  OutDataTypeStr=Inherit: Same as first input
  Switch : Switch  Commented=on  Criteria=u2 > Threshold
  Switch1 : Switch
  emission_in : Gain  Gain=emission_in  SaturateOnIntegerOverflow=on  OutDataTypeStr=Inherit: Same as input  ParamDataTypeStr=Inherit: Same as input
  heat flux downwards : Fcn  Expr=0.54*(abs(u(1)-u(2))^0.31)
  heat flux upwards : Fcn  Expr=2*(abs(u(1)-u(2))^0.31)
  lewis : Gain  Commented=on  Gain=0.000000007  SaturateOnIntegerOverflow=on  OutDataTypeStr=Inherit: Same as input  ParamDataTypeStr=Inherit: Same as input
  nomassflow : Constant  Value=0
  ps_l : Fcn  Commented=on  Expr=610.0*exp(17.08*(u)/(234.2+(u)))
  ps_s_l : Fcn  Commented=on  Expr=610.0*exp(17.08*(u)/(234.2+(u)))
  sigma : Constant  Value=5.67e-8
  view_factor : Gain  Gain=view_factor  SaturateOnIntegerOverflow=on  OutDataTypeStr=Inherit: Same as input  ParamDataTypeStr=Inherit: Same as input
  wallsurface : Gain  Gain=wallsurface  SaturateOnIntegerOverflow=on  OutDataTypeStr=Inherit: Same as input  ParamDataTypeStr=Inherit: Same as input
  wallsurface1 : Gain  Commented=on  Gain=wallsurface  SaturateOnIntegerOverflow=on  OutDataTypeStr=Inherit: Same as input  ParamDataTypeStr=Inherit: Same as input
  x2RelHum_UIBK : carnot/Basic/Material_Properties/x2RelHum  Commented=on
  qdots : Outport  InitialOutput=0
  "[S]" : Outport  Port=2  InitialOutput=0
  alpha_c : Outport  Port=3  InitialOutput=0
  phi_i_1/100 : Outport  Port=4  InitialOutput=0
  wires:
  nomassflow/1 -> Mux1/3, Switch/3
  wallsurface1/1 -> Switch/1
  view_factor/1 -> Product/1
  phis/1 -> Product3/1, Switch/2
  Add/1 -> lewis/1
  Product2/1 -> Add/2
  Product3/1 -> Add/1
  ps_s_l/1 -> Product3/2
  ps_l/1 -> Product2/2
  Constant/1 -> Mux1/2
  Constant1/1 -> Mux1/4
  Constant2/1 -> Mux1/5
  lewis/1 -> wallsurface1/1
  Gain2/1 -> Product2/1, phi_i_1/100/1
  Bus Selector/4 -> x2RelHum_UIBK/3  "<x_H2O>"
  Bus Selector/3 -> x2RelHum_UIBK/2  "<p>"
  x2RelHum_UIBK/1 -> Gain2/1
  Fcn1/1 -> Product/2
  Mux3/1 -> Fcn1/1
  sigma/1 -> emission_in/1
  Mux1/1 -> "[S]"/1
  Sum2/1 -> qdots/1
  AIB/1 -> Bus Selector/1
  Bus Selector/1 -> Sum/2, Mux2/2, x2RelHum_UIBK/1, ps_l/1  "<Tc>"
  emission_in/1 -> view_factor/1
  Product/1 -> Sum2/3, Mux/2  "qdotr"
  Mux/1 -> wallsurface/1
  Ts/1 -> Sum/1, ps_s_l/1, Mux3/1, Mux2/1  "Ts"
  Bus Selector/2 -> Mux3/2  "<Tr>"
  Mux2/1 -> heat flux downwards/1, heat flux upwards/1
  Product1/1 -> Mux/1, Sum2/2  "qdotc"
  Switch1/1 -> Product1/2, alpha_c/1  "hc"
  wallsurface/1 -> Mux1/1  "[Qdotc, Qdotr]"
  Qdot sol/1 -> 1/wallsurface/1
  1/wallsurface/1 -> Sum2/1
  Sum/1 -> Switch1/2, Product1/1  "dTc"
  heat flux upwards/1 -> Switch1/3
  heat flux downwards/1 -> Switch1/1

== system carnotUIBK/wall_zone/UA/Rse/AMBIENT ==
  WDB : Inport
  GDB : Inport  Port=2
  NDB : Inport  Port=3
  AIB : Inport  Port=4
  Qdot_sol : Inport  Port=5
  Qdot_in : Inport  Port=6
  R : Inport  Port=7
  Rsi : Inport  Port=8
  0.04 : Constant  Value=0.04
  0.13 : Constant  Value=0.13
  Bus Selector : BusSelector  OutputSignals=Temperature_Ambient
  Bus Selector1 : BusSelector  OutputSignals=Ts
  Constant : Constant  Value=zeros(1,5)
  Constant1 : Constant  Value=zeros(1,9)
  Constant2 : Constant  Value=zeros(1,1)
  Mux1 : Mux  Inputs=[1 1 5 1 9 1 1]
  Qdot : Sum  Inputs=3
  Qdot_T : Product  Inputs=**/
  Qdotr/Qdotc : Gain  Gain=0.5
  Rsum : Sum  Inputs=3
  Switch : Switch  Threshold=.75
  Terminator : Terminator
  Terminator1 : Terminator
  amb_factor : Constant  Value=amb_factor
  dT : Sum  Inputs=+-
  wallsurface : Constant  Value=wallsurface
  "[S]" : Outport
  wires:
  Constant/1 -> Mux1/3
  Qdot_in/1 -> Mux1/6, Qdot/3
  Qdot_sol/1 -> Qdot/2
  Qdot/1 -> Qdotr/Qdotc/1
  Qdot_T/1 -> Mux1/4, Qdot/1
  wallsurface/1 -> Qdot_T/2
  Rsum/1 -> Qdot_T/3
  dT/1 -> Qdot_T/1
  Bus Selector1/1 -> dT/2  "<Ts>"
  AIB/1 -> Bus Selector1/1
  Bus Selector/1 -> dT/1  "<Temperature_Ambient>"
  WDB/1 -> Bus Selector/1
  NDB/1 -> Terminator1/1
  GDB/1 -> Terminator/1
  Rsi/1 -> Rsum/3
  R/1 -> Rsum/2
  Qdotr/Qdotc/1 -> Mux1/1, Mux1/2
  Mux1/1 -> "[S]"/1
  amb_factor/1 -> Switch/2
  0.04/1 -> Switch/3
  0.13/1 -> Switch/1
  Switch/1 -> Rsum/1
  Constant1/1 -> Mux1/5
  Constant2/1 -> Mux1/7

== system carnotUIBK/wall_zone/UA/Rse/GROUND ==
  WDB : Inport
  GDB : Inport  Port=2
  NDB : Inport  Port=3
  AIB : Inport  Port=4
  Qdot_sol : Inport  Port=5
  Qdot_in : Inport  Port=6
  R : Inport  Port=7
  Rsi : Inport  Port=8
  0 : Constant  Value=0
  Add : Sum  Inputs=3
  Add1 : Sum  Inputs=+-
  Add2 : Sum  Inputs=3
  Bus Selector1 : BusSelector  OutputSignals=Ts
  Constant : Constant  Value=zeros(1,6)
  Constant1 : Constant  Value=zeros(1,8)
  Constant2 : Constant  Value=zeros(1,1)
  Mux1 : Mux  Inputs=[1 1 6 1 8 1 1]
  Qdot_T : Product  Inputs=**/
  Qdotr/Qdotc : Gain  Gain=0.5
  Terminator : Terminator
  Terminator1 : Terminator
  wallsurface : Constant  Value=wallsurface
  "[S]" : Outport
  wires:
  Qdot_sol/1 -> Add2/2
  Add2/1 -> Qdotr/Qdotc/1
  wallsurface/1 -> Qdot_T/2
  Add/1 -> Qdot_T/3
  Add1/1 -> Qdot_T/1
  Bus Selector1/1 -> Add1/2  "<Ts>"
  AIB/1 -> Bus Selector1/1
  WDB/1 -> Terminator/1
  NDB/1 -> Terminator1/1
  GDB/1 -> Add1/1
  Rsi/1 -> Add/3
  R/1 -> Add/2
  0/1 -> Add/1
  Qdotr/Qdotc/1 -> Mux1/1, Mux1/2
  Mux1/1 -> "[S]"/1
  Constant/1 -> Mux1/3
  Qdot_in/1 -> Mux1/6, Add2/3
  Qdot_T/1 -> Mux1/4, Add2/1
  Constant1/1 -> Mux1/5
  Constant2/1 -> Mux1/7

== system carnotUIBK/wall_zone/UA/Rse/INTERNAL ==
  WDB : Inport
  GDB : Inport  Port=2
  NDB : Inport  Port=3
  AIB : Inport  Port=4
  Qdot_sol : Inport  Port=5
  Qdot_in : Inport  Port=6
  R : Inport  Port=7
  Rsi : Inport  Port=8
  0.13 : Constant  Commented=on  Value=0.13
  Add : Sum  Commented=on  Inputs=3
  Add1 : Sum  Commented=on  Inputs=+-
  Add2 : Sum  Inputs=3
  Constant : Constant  Value=zeros(1,5)
  Constant1 : Constant  Value=zeros(1,9)
  Constant2 : Constant  Value=zeros(1,1)
  Constant3 : Constant  Value=zeros(1,1)
  Constant4 : Constant  Value=0
  Mux1 : Mux  Inputs=[1 1 5 1 9 1 1]
  Qdot_T : Product  Commented=on  Inputs=**/
  Qdotr/Qdotc : Gain  Gain=0.5
  Terminator{,1..3} (4 alike) : Terminator
  wallsurface : Constant  Commented=on  Value=wallsurface
  "[S]" : Outport
  wires:
  Qdot_sol/1 -> Add2/2
  Add2/1 -> Qdotr/Qdotc/1
  wallsurface/1 -> Qdot_T/2
  Add/1 -> Qdot_T/3
  Add1/1 -> Qdot_T/1
  AIB/1 -> Terminator3/1
  WDB/1 -> Terminator2/1
  NDB/1 -> Terminator1/1
  GDB/1 -> Terminator/1
  Rsi/1 -> Add/3
  R/1 -> Add/2
  0.13/1 -> Add/1
  Qdotr/Qdotc/1 -> Mux1/2, Mux1/1
  Mux1/1 -> "[S]"/1
  Constant/1 -> Mux1/3
  Qdot_in/1 -> Mux1/6, Add2/3
  Constant1/1 -> Mux1/5
  Constant2/1 -> Mux1/7
  Constant3/1 -> Mux1/4
  Constant4/1 -> Add2/1

== system carnotUIBK/wall_zone/UA/Rse/NEIGHBOUR ==
  WDB : Inport
  GDB : Inport  Port=2
  NDB : Inport  Port=3
  AIB : Inport  Port=4
  Qdot_sol : Inport  Port=5
  Qdot_in : Inport  Port=6
  R : Inport  Port=7
  Rsi : Inport  Port=8
  0.13 : Constant  Value=0.13
  Add : Sum  Inputs=3
  Add1 : Sum  Inputs=+-
  Add2 : Sum  Inputs=3
  Bus Selector1 : BusSelector  OutputSignals=Ts
  Constant : Constant  Value=zeros(1,7)
  Constant1 : Constant  Value=zeros(1,7)
  Constant2 : Constant  Value=zeros(1,1)
  Mux1 : Mux  Inputs=[1 1 7 1 7 1 1]
  Qdot_T : Product  Inputs=**/
  Qdotr/Qdotc : Gain  Gain=0.5
  Terminator : Terminator
  Terminator2 : Terminator
  wallsurface : Constant  Value=wallsurface
  "[S]" : Outport
  wires:
  Qdot_sol/1 -> Add2/2
  Add2/1 -> Qdotr/Qdotc/1
  wallsurface/1 -> Qdot_T/2
  Add/1 -> Qdot_T/3
  Add1/1 -> Qdot_T/1
  Bus Selector1/1 -> Add1/2  "<Ts>"
  AIB/1 -> Bus Selector1/1
  NDB/1 -> Add1/1
  GDB/1 -> Terminator/1
  Rsi/1 -> Add/3
  R/1 -> Add/2
  0.13/1 -> Add/1
  Qdotr/Qdotc/1 -> Mux1/1, Mux1/2
  Mux1/1 -> "[S]"/1
  Constant/1 -> Mux1/3
  Qdot_in/1 -> Mux1/6, Add2/3
  Qdot_T/1 -> Mux1/4, Add2/1
  Constant1/1 -> Mux1/5
  Constant2/1 -> Mux1/7
  WDB/1 -> Terminator2/1

== system carnotUIBK/wall_zone/UA/Rsi/down ==
  0.17 : Constant  Value=0.17
  Rsi : Outport
  wires:
  0.17/1 -> Rsi/1

== system carnotUIBK/wall_zone/UA/Rsi/horizontal ==
  0.13 : Constant  Value=0.13
  Rsi : Outport
  wires:
  0.13/1 -> Rsi/1

== system carnotUIBK/wall_zone/UA/Rsi/up ==
  0.10 : Constant  Value=0.10
  Rsi : Outport
  wires:
  0.10/1 -> Rsi/1

== system carnotUIBK/wall_zone/hygrothermal model/alpha_e/alpha_e_AMBIENT ==
  note: dynamic, convective heat transfer coefficients according to: Glück B.: Wärmeübergangskoeffizienten an thermisch aktiven Bauteiloberflächen
      | und der Übergang zu Basiskennlinien für die Wärmestromdichte; gi Gesundheits-Ingenieur; 128. Jahrgang 2007, Heft 1, Seiten 1-10
  note: Convective heat transfer outer surface according to EN 6946
      | Radiative heat transfer to the ground is limited by a view of 0.25, i.e. view factor to the sky is 0.75 (Frohner, 2005)
  note: s: surface
      | c: convective
      | r: radiative
      | h: in height
      | t: tilted surface
  note: CONVENTION:
      | qdots < 0, if Ts > T, heat flows from window surface (resp. room node) to ambient,
      | qdots > 0, if Ts < T, heat flows from ambient to window surface (resp. room node).
  WDB : Inport
  GDB : Inport  Port=2
  NDB : Inport  Port=3
  AIB : Inport  Port=4
  Ts : Inport  Port=5
  Qdot_sol : Inport  Port=6
  phis : Inport  Port=7
  1/100 : Gain  Gain=1/100
  Bus Selector : BusSelector  OutputSignals=Temperature_Ambient,Temperature_Sky_Radiation,Wind_Speed,Relative_Humidity
  Constant : Constant  Value=zeros(1,5)
  Constant1 : Constant  Value=zeros(1,2)
  Constant2 : Constant  Value=zeros(1,9)
  Mux1 : Mux  Inputs=[1 1 5 1 2 9]
  Product2 : Product  SaturateOnIntegerOverflow=on  RndMeth=Zero  InputSameDT=on  OutDataTypeStr=Inherit: Same as first input
  Qdotc : Constant  Value=0
  Qdotr : Constant  Value=0
  Sum : Sum  Inputs=+-  SaturateOnIntegerOverflow=on  InputSameDT=on  OutDataTypeStr=Inherit: Same as first input
  Sum2 : Sum  Inputs=+++  SaturateOnIntegerOverflow=on  InputSameDT=on  OutDataTypeStr=Inherit: Same as first input
  Terminator{,1..4} (5 alike) : Terminator
  absorption_out : Gain  Gain=absorption_out  SaturateOnIntegerOverflow=on  OutDataTypeStr=Inherit: Same as input  ParamDataTypeStr=Inherit: Same as input
  qp rad : Subsystem
  wall_surfrad : Subsystem  mask{pos=pos}
      mask prompts: pos "Position"
  wallsurface : Gain  Gain=wallsurface  SaturateOnIntegerOverflow=on  OutDataTypeStr=Inherit: Same as input  ParamDataTypeStr=Inherit: Same as input
  wind dependent heat transfer EN 6946 : Fcn  Expr=4*u(1)+4
  qdots : Outport  InitialOutput=0
  "[S]" : Outport  Port=2  InitialOutput=0
  alpha_c : Outport  Port=3  InitialOutput=0
  phi_e_1/100 : Outport  Port=4  InitialOutput=0
  theta_e : Outport  Port=5  InitialOutput=0
  wires:
  wallsurface/1 -> Mux1/4
  Sum2/1 -> qdots/1, wallsurface/1
  Qdotr/1 -> Mux1/2
  Qdotc/1 -> Mux1/1
  Constant/1 -> Mux1/3
  Constant1/1 -> Mux1/5
  Constant2/1 -> Mux1/6
  Mux1/1 -> "[S]"/1
  NDB/1 -> Terminator1/1
  GDB/1 -> Terminator/1
  Bus Selector/3 -> wind dependent heat transfer EN 6946/1  "<Wind_Speed>"
  Bus Selector/2 -> qp rad/3(Tsky)  "<Temperature_Sky_Radiation>"
  Bus Selector/1 -> theta_e/1, qp rad/1(Ta), Sum/1  "<Temperature_Ambient>"
  Sum/1 -> Product2/1  "dTc"
  WDB/1 -> wall_surfrad/1(WDB), Bus Selector/1
  Ts/1 -> Sum/2, qp rad/2(Tw)  "Ts (outer wall surface)"
  wall_surfrad/1(Idir,t+Idfu,t) -> absorption_out/1
  wind dependent heat transfer EN 6946/1 -> Product2/2, alpha_c/1  "alfa"
  absorption_out/1 -> Sum2/3  "qdot,sun"
  Product2/1 -> Sum2/1  "qdotc"
  qp rad/1(qprad) -> Sum2/2  "qdotr"
  AIB/1 -> Terminator2/1
  Qdot_sol/1 -> Terminator3/1
  phis/1 -> Terminator4/1
  Bus Selector/4 -> 1/100/1  "<Relative_Humidity>"
  1/100/1 -> phi_e_1/100/1

== system carnotUIBK/wall_zone/hygrothermal model/alpha_e/alpha_e_GROUND ==
  note: dynamic, convective heat transfer coefficients according to: Glück B.: Wärmeübergangskoeffizienten an thermisch aktiven Bauteiloberflächen
      | und der Übergang zu Basiskennlinien für die Wärmestromdichte; gi Gesundheits-Ingenieur; 128. Jahrgang 2007, Heft 1, Seiten 1-10
  note: Convective heat transfer outer surface according to EN 6946
      | Radiative heat transfer to the ground is limited by a view of 0.25, i.e. view factor to the sky is 0.75 (Frohner, 2005)
  note: s: surface
      | c: convective
      | r: radiative
      | h: in height
      | t: tilted surface
  note: CONVENTION:
      | qdots < 0, if Ts > T, heat flows from window surface (resp. room node) to ambient,
      | qdots > 0, if Ts < T, heat flows from ambient to window surface (resp. room node).
  WDB : Inport
  GDB : Inport  Port=2
  NDB : Inport  Port=3
  AIB : Inport  Port=4
  Ts : Inport  Port=5
  Qdot_sol : Inport  Port=6
  phis : Inport  Port=7
  Constant : Constant  Value=zeros(1,5)
  Constant1 : Constant  Value=0
  Constant2 : Constant  Value=zeros(1,10)
  Mux1 : Mux  Inputs=[1 1 5 1 1 10]
  Qdotc : Constant  Value=0
  Qdotr : Constant  Value=0
  Sum : Sum  Inputs=+-  SaturateOnIntegerOverflow=on  InputSameDT=on  OutDataTypeStr=Inherit: Same as first input
  Terminator{,1..4} (5 alike) : Terminator
  alpha1000 : Constant  Value=1000
  alpha_ground : Gain  Gain=1000
  phi100 : Constant
  wallsurface : Gain  Gain=wallsurface  SaturateOnIntegerOverflow=on  OutDataTypeStr=Inherit: Same as input  ParamDataTypeStr=Inherit: Same as input
  qdots : Outport  InitialOutput=0
  "[S]" : Outport  Port=2  InitialOutput=0
  alpha_c : Outport  Port=3  InitialOutput=0
  phi_e_1/100 : Outport  Port=4  InitialOutput=0
  theta_e : Outport  Port=5  InitialOutput=0
  wires:
  alpha_ground/1 -> qdots/1, wallsurface/1
  Qdotr/1 -> Mux1/2
  Qdotc/1 -> Mux1/1
  Constant/1 -> Mux1/3
  Constant2/1 -> Mux1/6
  Mux1/1 -> "[S]"/1
  NDB/1 -> Terminator1/1
  GDB/1 -> theta_e/1, Sum/1
  Sum/1 -> alpha_ground/1  "dT"
  Ts/1 -> Sum/2  "Ts (outer wall surface)"
  AIB/1 -> Terminator2/1
  WDB/1 -> Terminator/1
  Qdot_sol/1 -> Terminator3/1
  phis/1 -> Terminator4/1
  phi100/1 -> phi_e_1/100/1
  alpha1000/1 -> alpha_c/1
  Constant1/1 -> Mux1/4
  wallsurface/1 -> Mux1/5

== system carnotUIBK/wall_zone/hygrothermal model/alpha_e/alpha_e_INTERNAL ==
  note: dynamic, convective heat transfer coefficients according to: Glück B.: Wärmeübergangskoeffizienten an thermisch aktiven Bauteiloberflächen
      | und der Übergang zu Basiskennlinien für die Wärmestromdichte; gi Gesundheits-Ingenieur; 128. Jahrgang 2007, Heft 1, Seiten 1-10
  note: Convective heat transfer outer surface according to EN 6946
      | Radiative heat transfer to the ground is limited by a view of 0.25, i.e. view factor to the sky is 0.75 (Frohner, 2005)
  note: s: surface
      | c: convective
      | r: radiative
      | h: in height
      | t: tilted surface
  note: CONVENTION:
      | qdots < 0, if Ts > T, heat flows from window surface (resp. room node) to ambient,
      | qdots > 0, if Ts < T, heat flows from ambient to window surface (resp. room node).
  WDB : Inport
  GDB : Inport  Port=2
  NDB : Inport  Port=3
  AIB : Inport  Port=4
  Ts : Inport  Port=5
  Qdot_sol : Inport  Port=6
  phis : Inport  Port=7
  Bus Selector : BusSelector  OutputSignals=Tc
  Terminator : Terminator
  Terminator1 : Terminator
  Terminator2 : Terminator
  alpha_i : Subsystem  Variant=on  mask{view_factor=amb_factor}
  qdots : Outport  InitialOutput=0
  "[S]" : Outport  Port=2  InitialOutput=0
  alpha_c : Outport  Port=3  InitialOutput=0
  phi_e_1/100 : Outport  Port=4  InitialOutput=0
  theta_e : Outport  Port=5  InitialOutput=0
  wires:
  NDB/1 -> Terminator1/1
  GDB/1 -> Terminator/1
  WDB/1 -> Terminator2/1
  Ts/1 -> alpha_i/1(Ts)  "Ts (outer wall surface)"
  Qdot_sol/1 -> alpha_i/3(Qdot sol)
  alpha_i/1(qdots) -> qdots/1
  alpha_i/3(alpha_c) -> alpha_c/1
  alpha_i/2("[S]") -> "[S]"/1
  AIB/1 -> alpha_i/2(AIB), Bus Selector/1
  phis/1 -> alpha_i/4(phis)
  alpha_i/4(phi_i_1/100) -> phi_e_1/100/1
  Bus Selector/1 -> theta_e/1  "<Tc>"

== system carnotUIBK/wall_zone/hygrothermal model/alpha_e/alpha_e_NEIGHBOUR ==
  note: dynamic, convective heat transfer coefficients according to: Glück B.: Wärmeübergangskoeffizienten an thermisch aktiven Bauteiloberflächen
      | und der Übergang zu Basiskennlinien für die Wärmestromdichte; gi Gesundheits-Ingenieur; 128. Jahrgang 2007, Heft 1, Seiten 1-10
  note: Convective heat transfer outer surface according to EN 6946
      | Radiative heat transfer to the ground is limited by a view of 0.25, i.e. view factor to the sky is 0.75 (Frohner, 2005)
  note: s: surface
      | c: convective
      | r: radiative
      | h: in height
      | t: tilted surface
  note: CONVENTION:
      | qdots < 0, if Ts > T, heat flows from window surface (resp. room node) to ambient,
      | qdots > 0, if Ts < T, heat flows from ambient to window surface (resp. room node).
  WDB : Inport
  GDB : Inport  Port=2
  NDB : Inport  Port=3
  AIB : Inport  Port=4
  Ts : Inport  Port=5
  Qdot_sol : Inport  Port=6
  phis : Inport  Port=7
  Demux : Demux  Outputs=[2 5 1 1 10]
  Mux1 : Mux  Inputs=[1 1 5 1 1 10]
  Qdot sol neighbour : Constant  Value=0
  Qdot_T_opaque : Constant  Value=0
  Qdotc : Constant  Value=0
  Qdotr : Constant  Value=0
  Terminator{,1..4} (5 alike) : Terminator
  alpha_i : Subsystem  Variant=on  mask{view_factor=1}
  set temperature : BusAssignment  AssignedSignals=Ts,Tc,Tr
  qdots : Outport  InitialOutput=0
  "[S]" : Outport  Port=2  InitialOutput=0
  alpha_c : Outport  Port=3  InitialOutput=0
  phi_e_1/100 : Outport  Port=4  InitialOutput=0
  theta_e : Outport  Port=5  InitialOutput=0
  wires:
  GDB/1 -> Terminator/1
  WDB/1 -> Terminator2/1
  Ts/1 -> alpha_i/1(Ts)  "Ts (outer wall surface)"
  alpha_i/1(qdots) -> qdots/1
  alpha_i/3(alpha_c) -> alpha_c/1
  phis/1 -> alpha_i/4(phis)
  alpha_i/4(phi_i_1/100) -> phi_e_1/100/1
  Qdot_sol/1 -> Terminator3/1
  Qdot sol neighbour/1 -> alpha_i/3(Qdot sol)
  AIB/1 -> set temperature/1
  NDB/1 -> theta_e/1, set temperature/4, set temperature/3, set temperature/2
  set temperature/1 -> alpha_i/2(AIB)
  alpha_i/2("[S]") -> Demux/1
  Demux/1 -> Terminator1/1
  Qdotr/1 -> Mux1/2
  Qdotc/1 -> Mux1/1
  Demux/2 -> Mux1/3
  Demux/5 -> Mux1/6
  Mux1/1 -> "[S]"/1
  Qdot_T_opaque/1 -> Mux1/4
  Demux/3 -> Terminator4/1
  Demux/4 -> Mux1/5
